simulink model "evirici_3faz"  (R2017a)
settings: Solver=ode15s  StartTime=0.0  StopTime=0.1  RelTol=1e-3  EnableMultiTasking=on
libraries: powerlib x13, powerlib_meascontrol x2
settings Model: Creator=hp  LastModifiedBy=HCS
settings DataIOCC: LimitDataPoints=on  SaveFormat=Array  SignalLoggingSaveFormat=ModelDataLogs
settings OptimizationCC: ExpressionDepthLimit=2147483647  InitFltsAndDblsToZero=on  LifeSpan=inf
settings DebuggingCC: SaveWithParameterizedLinksMsg=none  UnderspecifiedInitializationDetection=Classic  MergeDetectMultiDrivingBlocksExec=none  SignalResolutionControl=TryResolveAllWithWarning  SolverPrmCheckMsg=warning  MultiTaskDSMMsg=warning  MultiTaskCondExecSysMsg=none  FcnCallInpInsideContextMsg=warning  StateNameClashWarn=warning  SFUnexpectedBacktrackingDiag=warning  SFNoUnconditionalDefaultTransitionDiag=warning  SFExecutionAtInitializationDiag=none
settings HardwareCC: ProdBitPerPointer=32  ProdBitPerSizeT=32  ProdBitPerPtrDiffT=32  ProdLargestAtomicFloat=None  ProdIntDivRoundTo=Undefined  ProdEndianess=Unspecified  ProdWordSize=32  ProdHWDeviceType=32-bit Generic
settings ModelReferenceCC: PropagateSignalLabelsOutOfModel=off
settings GRTTargetCC: TargetFcnLib=ansi_tfl_tmw.mat  TargetLangStandard=C89/C90 (ANSI)  CombineOutputUpdateFcns=off  GRTInterface=on
settings ConfigComp: CovMetricSettings=dw  CovSaveCumulativeToWorkspaceVar=on  CovSaveSingleToWorkspaceVar=on  CovExternalEMLEnable=off
settings SimscapeCC: SimscapeNormalizeSystem=off

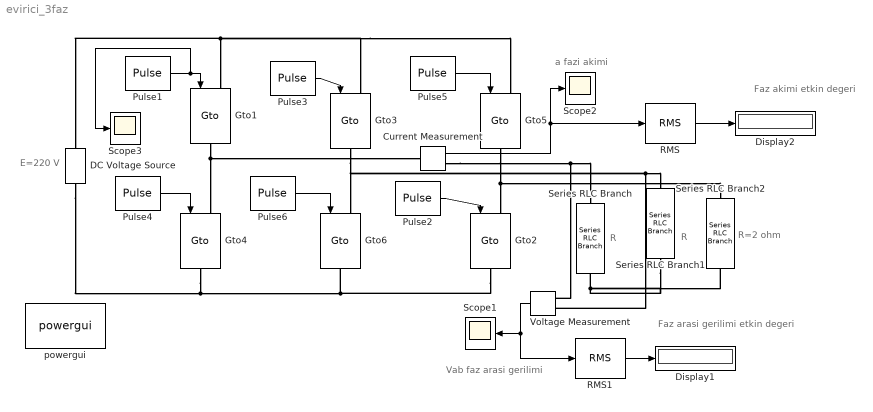
== system evirici_3faz ==
  note: R
  note: R
  note: R=2 ohm
  note: a fazi akimi
  note: Vab faz arasi
      | gerilimi
  note: E=220 V
  note: Faz arasi gerilimi
      | etkin degeri
  note: Faz akimi
      | etkin degeri
  Current Measurement : powerlib/Measurements/Current Measurement  PhasorSimulation=off  OutputType=Complex  PSBequivalent=0
  DC Voltage Source : powerlib/Electrical Sources/DC Voltage Source  Amplitude=220  Measurements=None
  Display1 : Display
  Display2 : Display
  Gto{1..6} (6 alike) : powerlib/Power Electronics/Gto  Ron=0.001  Lon=1e-6  Vf=1  Tf=10e-6  Tt=20e-6  IC=0  Rs=1e5  Cs=inf  Measurements=off
      settings: SourceProductBaseCode=PS
  Pulse1 : DiscretePulseGenerator  PulseType=Time based  Period=0.02  PulseWidth=100*(120/360)
  Pulse2 : DiscretePulseGenerator  PulseType=Time based  Period=0.02  PulseWidth=100*(120/360)  PhaseDelay=0.02/6
  Pulse3 : DiscretePulseGenerator  PulseType=Time based  Period=0.02  PulseWidth=100*(120/360)  PhaseDelay=2*(0.02/6)
  Pulse4 : DiscretePulseGenerator  PulseType=Time based  Period=0.02  PulseWidth=100*(120/360)  PhaseDelay=3*(0.02/6)
  Pulse5 : DiscretePulseGenerator  PulseType=Time based  Period=0.02  PulseWidth=100*(120/360)  PhaseDelay=4*(0.02/6)
  Pulse6 : DiscretePulseGenerator  PulseType=Time based  Period=0.02  PulseWidth=100*(120/360)  PhaseDelay=5*(0.02/6)
  RMS : powerlib_meascontrol/Measurements/RMS  TrueRMS=on  Freq=50  RMSInit=100  Ts=0
  RMS1 : powerlib_meascontrol/Measurements/RMS  TrueRMS=on  Freq=50  RMSInit=100  Ts=0
  Scope1 : Scope
  Scope2 : Scope
  Scope3 : Scope
  Series RLC Branch : powerlib/Elements/Series RLC Branch  LConnTagsString=__new0  RConnTagsString=__new0  BranchType=R  Resistance=2  Inductance=0  SetiL0=off  InitialCurrent=0  Capacitance=inf  Setx0=off  InitialVoltage=0  Measurements=None
  Series RLC Branch1 : powerlib/Elements/Series RLC Branch  LConnTagsString=__new0  RConnTagsString=__new0  BranchType=R  Resistance=2  Inductance=0  SetiL0=off  InitialCurrent=0  Capacitance=inf  Setx0=off  InitialVoltage=0  Measurements=None
  Series RLC Branch2 : powerlib/Elements/Series RLC Branch  LConnTagsString=__new0  RConnTagsString=__new0  BranchType=R  Resistance=2  Inductance=0  SetiL0=off  InitialCurrent=0  Capacitance=inf  Setx0=off  InitialVoltage=0  Measurements=None
  Voltage Measurement : powerlib/Measurements/Voltage Measurement  PhasorSimulation=off  OutputType=Complex  PSBequivalent=0
  powergui : powerlib/powergui  Priority=2  SimulationMode=Discrete  SampleTime=50e-6  frequency=50  Iterations=50  frequencyindice=0  Pbase=100e6  ErrMax=1e-4  UnitsV=kV  UnitsW=MW  buscounter=0  FunctionMessages=off  echomessages=off  EnableUseOfTLC=off  CurrentSourceSwitches=off  DisableSnubberDevices=off  DisableRonSwitches=off  DisableVfSwitches=off  DisplayEquations=off  AutomaticDiscreteSolvers=off  SolverType=Tustin  Interpol=off  ExternalGateDelay=off  methode=off  Ts=0  x0status=blocks  SPID=off  SwTol=0  HookPort=off  NonlinearTolerance=1e-4  nMaxIteration=100  ContinueOnMaxIteration=off  RestoreLinks=warning  ResistiveCurrentMeasurement=off  Frange=[0:2:500]  Ylog=off  Xlog=on  ShowGrid=off  save=off  variable=ZData  structure=ScopeData  ZoomFFT=on  StartTime=0.0  cycles=1  DisplayStyle=1  fundamental=50  FreqAxis=off  MaxFrequency=1000  frequencyindicesteady=1  RmsSteady=1  display=off
  wires:
  Pulse1/1 -> Gto1/1, Scope3/1
  Pulse3/1 -> Gto3/1
  Pulse5/1 -> Gto5/1
  Pulse4/1 -> Gto4/1
  Pulse6/1 -> Gto6/1
  Pulse2/1 -> Gto2/1
  Current Measurement/1 -> RMS/1, Scope2/1
  Voltage Measurement/1 -> RMS1/1, Scope1/1
  RMS1/1 -> Display1/1
  RMS/1 -> Display2/1
  connections:
  Series RLC Branch/RConn1 -- Series RLC Branch2/RConn1 -- Series RLC Branch1/RConn1
  Gto3/LConn1 -- Gto5/LConn1 -- DC Voltage Source/RConn1 -- Gto1/LConn1
  DC Voltage Source/LConn1 -- Gto6/RConn1 -- Gto2/RConn1 -- Gto4/RConn1
  Gto1/RConn1 -- Gto4/LConn1 -- Current Measurement/LConn1
  Gto3/RConn1 -- Gto6/LConn1 -- Series RLC Branch1/LConn1 -- Voltage Measurement/LConn2
  Gto5/RConn1 -- Gto2/LConn1 -- Series RLC Branch2/LConn1
  Current Measurement/RConn1 -- Series RLC Branch/LConn1 -- Voltage Measurement/LConn1
